simulink model "vChassis"  (R2024b)
settings: Solver=FixedStepAuto  StartTime=0.0  StopTime=10.0  RelTol=1e-3  EnableMultiTasking=on
undefined symbols (not defined in the file): tSystemsTask
settings Model: DataDictionary=Master_Dictionary.sldd  EnableAccessToBaseWorkspace=off  Creator=torni  LastModifiedBy=Will
settings OptimizationCC: DefaultParameterBehavior=Inlined  EnhancedBackFolding=on  PassReuseOutputArgsAs=Individual arguments  ZeroExternalMemoryAtStartup=off  ZeroInternalMemoryAtStartup=off  MaxStackSize=8192  OptimizeBlockOrder=speed  DifferentSizesBufferReuse=on  OptimizationCustomize=off  EfficientTunableParamExpr=on
settings DebuggingCC: ParameterTunabilityLossMsg=error
settings HardwareCC: ProdBitPerPointer=32  ProdBitPerSizeT=32  ProdBitPerPtrDiffT=32  ProdLargestAtomicInteger=Long  ProdLargestAtomicFloat=Double  ProdWordSize=32  ProdLongLongMode=on  ProdHWDeviceType=ARM Compatible->ARM Cortex-M
settings SFSimCC: MATLABDynamicMemAlloc=off
settings RTWCC: Description=Embedded Coder  SystemTargetFile=ert.tlc  HardwareBoard=STM32H7xx Based (Single-core)  TemplateMakefile=ert_default_tmf  Toolchain=GNU Tools for ARM Embedded Processors
settings CodeAppCC: ForceParamTrailComments=on  IgnoreCustomStorageClasses=off  OperatorAnnotations=on  SimulinkDataObjDesc=on  SFDataObjDesc=on  InsertBlockDesc=on
settings ERTTargetCC: TargetLangStandard=C99 (ISO)  CodeReplacementLibrary=ARM Cortex-M  ExtModeTransport=3  ExtModeStaticAlloc=on  ExtModeStaticAllocSize=2048  ExtModeMexFile=ext_xcp  ExtModeIntrfLevel=Level2 - Open

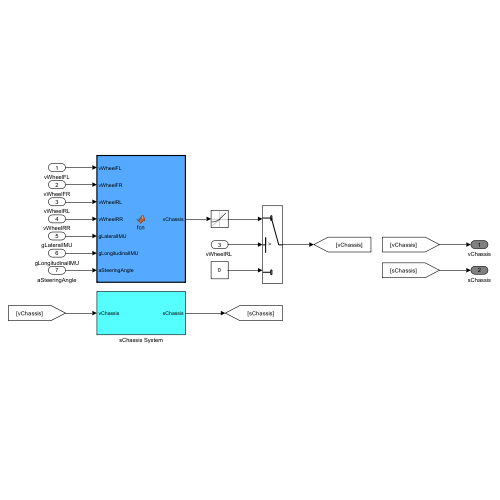
[thumbnail: Simulink's stored preview of the top-level diagram]
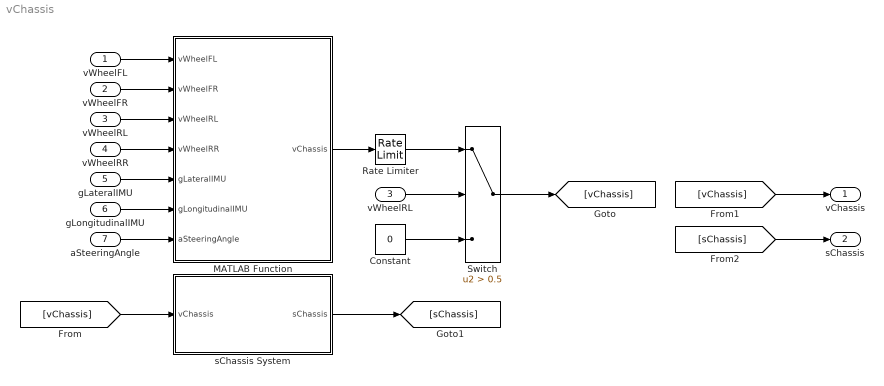
== system vChassis ==
  vWheelFL : Inport  OutDataTypeStr=double
  vWheelFR : Inport  Port=2  OutDataTypeStr=double
  vWheelRL : Inport  Port=3
  vWheelRR : Inport  Port=4
  gLateralIMU : Inport  Port=5
  gLongitudinalIMU : Inport  Port=6
  aSteeringAngle : Inport  Port=7
  Constant : Constant  Value=0
  MATLAB Function : MATLAB Function  TreatAsAtomicUnit=on
  Rate Limiter : RateLimiter  RisingSlewLimit=21.58  FallingSlewLimit=-21.58  SampleTimeMode=inherited
  Switch : Switch  Criteria=u2 > Threshold  Threshold=0.5  SaturateOnIntegerOverflow=off  InputSameDT=off
  sChassis System : Subsystem
  "vWheelRL " : InportShadow  Port=3
  vChassis : Outport  OutDataTypeStr=double  VectorParamsAs1DForOutWhenUnconnected=off
  sChassis : Outport  Port=2  OutDataTypeStr=double  VectorParamsAs1DForOutWhenUnconnected=off
  wires:
  aSteeringAngle/1 -> MATLAB Function/7(aSteeringAngle)
  gLongitudinalIMU/1 -> MATLAB Function/6(gLongitudinalIMU)
  vWheelRR/1 -> MATLAB Function/4(vWheelRR)
  gLateralIMU/1 -> MATLAB Function/5(gLateralIMU)
  vWheelRL/1 -> MATLAB Function/3(vWheelRL)
  [vChassis] -> vChassis/1
  vWheelFL/1 -> MATLAB Function/1(vWheelFL)
  Switch/1 -> [vChassis]
  [vChassis] -> sChassis System/1(vChassis)
  vWheelFR/1 -> MATLAB Function/2(vWheelFR)
  sChassis System/1(sChassis) -> [sChassis]
  [sChassis] -> sChassis/1
  MATLAB Function/1(vChassis) -> Rate Limiter/1
  "vWheelRL "/1 -> Switch/2
  Constant/1 -> Switch/3
  Rate Limiter/1 -> Switch/1

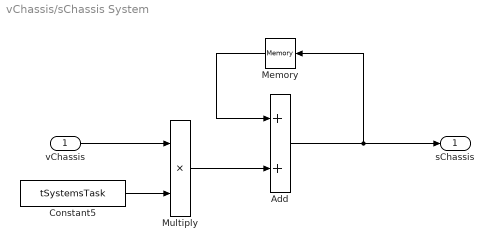
== system vChassis/sChassis System ==
  vChassis : Inport  OutDataTypeStr=double
  Add : Sum
  Constant5 : Constant  Value=tSystemsTask
  Memory : Memory  InheritSampleTime=on
  Multiply : Product
  sChassis : Outport  OutDataTypeStr=double  VectorParamsAs1DForOutWhenUnconnected=off
  wires:
  Multiply/1 -> Add/2
  Constant5/1 -> Multiply/2
  Memory/1 -> Add/1
  vChassis/1 -> Multiply/1
  Add/1 -> sChassis/1, Memory/1

== matlab function vChassis/MATLAB Function ==
  data: vWheelFL input; vWheelFR input; vChassis output; vWheelRL input; vWheelRR input; gLateralIMU input; gLongitudinalIMU input; aSteeringAngle input
%OBR24 vChassis Code:
function vChassis = fcn(vWheelFL, vWheelFR, vWheelRL, vWheelRR, gLateralIMU, gLongitudinalIMU, aSteeringAngle)

% VEHICLE PARAMETERS
Track = 1.23;     % meters
Tyre_out_diam = 406/1000;     % meters 

% Storing the angular velocities from T
w_FL = vWheelFL;
w_FR = vWheelFR;
w_RL = vWheelRL;
w_RR = vWheelRR;

% Storing other car parameters from T
ay = gLateralIMU;
ax = gLongitudinalIMU;
steer = aSteeringAngle;     % rad (POSITIVE = turning left)


% DEADZONE FOR THE STEERING
DEADZONE   = 3;     % DEG
BOOL  = [1 1 1 1];  % 1 if valid
% FL FR RL RR

% INITIALIZING
w_avg =  0;
R = 0;
v_est_acker = 0;

% acceptable range to predict tyres slipping or blocking
margin = 0.1; % 10% 
margin_turn = 0.1; % 10%


%  STRAIGHT LINE CONDITION
if abs(steer) < DEADZONE     
    if ax >= 0 % using rear for acceleration
        w_ref = (w_RL + w_RR) / 2;
        if abs(w_ref) < 0.65 % to avoid divide by zero
            w_avg = max([w_FL,w_FR,w_RL,w_RR]);
        else
            w_avg = w_ref;

            % RL
            if abs((w_avg-w_RL)/w_avg)>(margin)
                BOOL(3)=0;
            end
            
            % RR
            if abs((w_avg-w_RR)/w_avg)>(margin)
                BOOL(4)=0;
            end
            
            denom = BOOL(3) + BOOL(4);
            if denom > 0
                w_avg = (w_RL*BOOL(3) + w_RR*BOOL(4)) / denom;
            else
                w_avg = min([w_FL,w_FR,w_RL,w_RR]);
            end
        end
        
    else % using front for deceleration
        w_ref = (w_FL + w_FR) / 2;
  
        if abs(w_ref) < 0.65 % to avoid divide by zero
            w_avg = max([w_FL,w_FR,w_RL,w_RR]);
        else
            w_avg = w_ref;
    
            % FL
            if abs((w_avg-w_FL)/w_avg)>(margin)
                BOOL(1)=0;
            end
            
            % FR
            if abs((w_avg-w_FR)/w_avg)>(margin) 
                BOOL(2)=0;
            end
            
            denom = BOOL(1) + BOOL(2);
            if denom > 0
                w_avg = (w_FL*BOOL(1) + w_FR*BOOL(2)) / denom;
            else
                w_avg = max([w_FL,w_FR,w_RL,w_RR]);
            end
        end
    end

%  TURNING LEFT
elseif steer > 0

    if ax == 0
        w_avg = (w_FR + w_RR) / 2;
    elseif ax > 0
        w_avg = min(w_FR, w_RR);
    else
        w_avg = max(w_FR, w_RR);
    end


%  TURNING RIGHT
else

    if ax == 0
        w_avg = (w_FL + w_RL) / 2;
    elseif ax > 0
        w_avg = min(w_FL, w_RL);
    else
        w_avg = max(w_FL, w_RL);
    end
end


%  ACKERMANN CORRECTION
v_est = w_avg;

if abs(steer) > DEADZONE && abs(ay) > 1e-6
    R_i   = v_est^2 / abs(ay);
    R_cog = R_i - Track/2;
    vChassis = v_est * (R_cog / R_i);
else
    vChassis = v_est;
end

end
